simulink model "SG_RaibertControlMonopod"  (R2022a)
settings: Solver=ode4  StartTime=0.0  StopTime=inf  FixedStep=1/4000  MaxStep=0.001  RelTol=1e-3  AbsTol=1e-3  EnableMultiTasking=on
values from neighbouring files (symbols this model uses):
  alternate_legs = InitConstants.alternate_legs    [Controller.m]    (also in ControllerV2.m; ControllerV3.m; Controller_original.m; initialization.m = 1)
  dphi_IC = InitConstants.dphi_IC    [Controller.m]    (also in ControllerV2.m; ControllerV3.m; Controller_original.m; initialization.m = 0)
  dphi_RC_14 = 0.0    (= 0)    [initialization.m]
  dphi_RC_23 = 0.0    (= 0)    [initialization.m]
  dr_contact = -0.2    [initialization.m]
  dr_IC = InitConstants.dr_IC    [Controller.m]    (also in ControllerV2.m; ControllerV3.m; Controller_original.m; initialization.m = 0)
  dr_RC_14 = 0.0    (= 0)    [initialization.m]
  dr_RC_23 = 0.0    (= 0)    [initialization.m]
  dx_des = -InitConstants.dx_des    [Controller.m]    (also in ControllerV2.m; ControllerV3.m; Controller_original.m; Hopper_raibert_controller.m = -min(max(1.0*(x_body - x_des), -0.5), 0.5))
  Fthrust_RC_14 = 100    [initialization.m]
  Fthrust_RC_23 = 150    [initialization.m]
  GAIN_dx_RC_14 = 0.07    [initialization.m]
  GAIN_dx_RC_23 = 0.05    [initialization.m]
  Kd_phi_IC = InitConstants.Kd_phi_IC    [Controller.m]    (also in ControllerV2.m; ControllerV3.m; Controller_original.m; initialization.m = 15)
  Kd_phi_RC_14 = Kp_phi_RC_14*0.1    (= 10)    [initialization.m]
  Kd_phi_RC_23 = 15    [initialization.m]
  Kd_r_IC = InitConstants.Kd_r_IC    [Controller.m]    (also in ControllerV2.m; ControllerV3.m; Controller_original.m; initialization.m = 60)
  Kd_r_RC_14 = Kp_r_RC_14*0.1    (= 60)    [initialization.m]
  Kd_r_RC_23 = 150    [initialization.m]
  knee_limit = 160    [initialization.m]
  Kp_phi_IC = InitConstants.Kp_phi_IC    [Controller.m]    (also in ControllerV2.m; ControllerV3.m; Controller_original.m; initialization.m = 100)
  Kp_phi_RC_14 = 100    [initialization.m]
  Kp_phi_RC_23 = 100    [initialization.m]
  Kp_r_IC = InitConstants.Kp_r_IC    [Controller.m]    (also in ControllerV2.m; ControllerV3.m; Controller_original.m; initialization.m = 500)
  Kp_r_RC_14 = 600    [initialization.m]
  Kp_r_RC_23 = 600    [initialization.m]
  m_eff = 5    [ControllerV2.m]    (also in Controller_original.m; initialization.m)
  match_leg_gains = -1    [initialization.m]
  offset_phi_limit = 30    [initialization.m]
  phi_IC = InitConstants.phi_IC    [Controller.m]    (also in ControllerV2.m; ControllerV3.m; Controller_original.m; initialization.m = 0)
  phi_RC_14 = -0.003    [initialization.m]
  phi_RC_23 = -0.006    [initialization.m]
  r_IC = InitConstants.r_IC    [Controller.m]    (also in ControllerV2.m; ControllerV3.m; Controller_original.m; initialization.m = 0.32)
  r_RC_14 = 0.32    [initialization.m]
  r_RC_23 = 0.33    [initialization.m]
  r_thrust_RC_14 = 0.27    [initialization.m]
  r_thrust_RC_23 = 0.29    [initialization.m]
  tau_limit = 100    [initialization.m]
  update_controller_Kd_r = 1    [initialization.m]
  x_des = InitConstants.x_des    [Controller.m]    (also in ControllerV2.m; ControllerV3.m; Controller_original.m; initialization.m = 0)
undefined symbols (not defined in the file or in its folder): HS, IO291
libraries: speedgoatlib_IO691 x7, canmsglib x5, aru_toolbox x2, simulink x2, speedgoatlib_IO291 x1
(part 2 of 2)

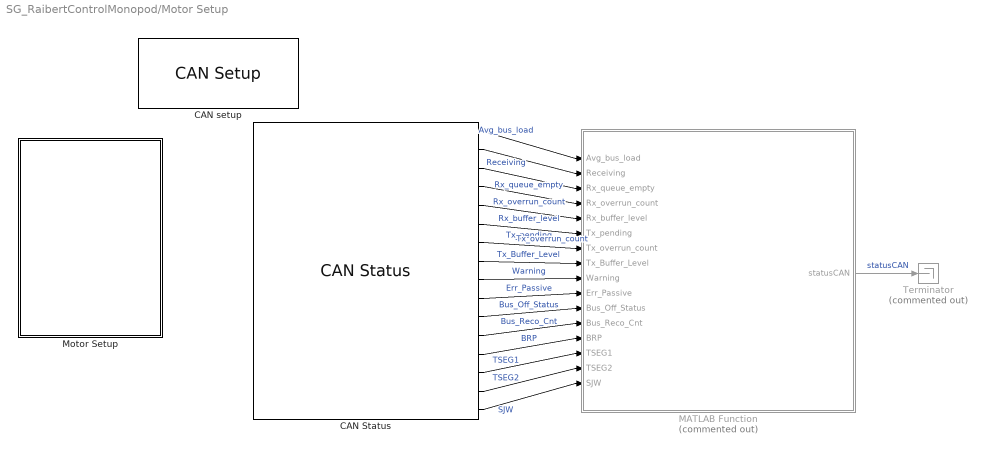
== system SG_RaibertControlMonopod/Motor Setup ==
  CAN Status : speedgoatlib_IO691/Legacy/CAN Status  moduleId=1  sampleTime=-1  channel=1  busRecovery=Off  arrayOutput=off  controllerCpuLoad=off  controllerLiveCount=off  initModeAct=off  avgBusLoad=on  receiving=on  RxQueueEmpty=on  dataOverrunRcv=on  rxBufferLevel=on  txPending=on  dataOverrunTx=on  txBufferLevel=on  errWarnLimit=on  errPassLimit=on  errBusOff=on  busRecoveryCounter=on  busCouplingErr=off  transceiverErr=off  opMode=off  brp=on  timeSegment1=on  timeSegment2=on  synchronisationJumpWidth=on  dataTSEG1=off  dataTSEG2=off  dataSJW=off  moduleType=691  qtyStatBlk=1  ptIdx=0  isFDMod=0
      settings: SourceProductName=Simulink Real-Time: Speedgoat I/O Blockset
  CAN setup : speedgoatlib_IO691/Legacy/CAN Setup   moduletype=IO691  id=1  pciSlot=-1  chn1=CAN (HS)  chn2=Disabled  chn3=Disabled  chn4=Disabled  initStruct=[]  termStruct=[struct('Channel',1,'Protocol','CAN','BRS',0,'Type','Standard','Identifier',2,'Data',[255, 255, 255, 255, 255, 255, 255, 253],'Pause',0.001), struct('Channel',1,'Protocol','CAN','BRS',0,'Type','Standard','Identifier',3,'Data',[255, 255, 255, 255, 255, 255, 255, 253],'Pause',0.001)]  ArbitrationbdrChn1=1.0 MBaud  ArbitrationManbdrChn1=[2,8,31,8]  FdbdrChn1=1.0 MBaud  FdManbdrChn1=[2,8,31,8]  ArbitrationbdrChn2=1.0 MBaud  ArbitrationManbdrChn2=[2,8,31,8]  FdbdrChn2=1.0 MBaud  FdManbdrChn2=[2,8,31,8]  ArbitrationbdrChn3=1.0 MBaud  ArbitrationManbdrChn3=[2,8,31,8]  FdbdrChn3=5.0 MBaud  FdManbdrChn3=[2,2,5,2]  ArbitrationbdrChn4=1.0 MBaud  ArbitrationManbdrChn4=[2,8,31,8]  FdbdrChn4=5.0 MBaud  FdManbdrChn4=[2,2,5,2]  moduleInitValues=[691 1 -1 -1]
      settings: SourceProductName=Simulink Real-Time: Speedgoat I/O Blockset
  MATLAB Function : MATLAB Function  Commented=on  TreatAsAtomicUnit=on
  Motor Setup : Subsystem
  Terminator : Terminator  Commented=on
  wires:
  CAN Status/1 -> MATLAB Function/1(Avg_bus_load)  "Avg_bus_load"
  CAN Status/2 -> MATLAB Function/2(Receiving)  "Receiving"
  CAN Status/3 -> MATLAB Function/3(Rx_queue_empty)  "Rx_queue_empty"
  CAN Status/4 -> MATLAB Function/4(Rx_overrun_count)  "Rx_overrun_count"
  CAN Status/5 -> MATLAB Function/5(Rx_buffer_level)  "Rx_buffer_level"
  CAN Status/6 -> MATLAB Function/6(Tx_pending)  "Tx_pending"
  CAN Status/8 -> MATLAB Function/8(Tx_Buffer_Level)  "Tx_Buffer_Level"
  CAN Status/7 -> MATLAB Function/7(Tx_overrun_count)  "Tx_overrun_count"
  CAN Status/12 -> MATLAB Function/12(Bus_Reco_Cnt)  "Bus_Reco_Cnt"
  CAN Status/13 -> MATLAB Function/13(BRP)  "BRP"
  CAN Status/15 -> MATLAB Function/15(TSEG2)  "TSEG2"
  CAN Status/14 -> MATLAB Function/14(TSEG1)  "TSEG1"
  CAN Status/10 -> MATLAB Function/10(Err_Passive)  "Err_Passive"
  CAN Status/9 -> MATLAB Function/9(Warning)  "Warning"
  CAN Status/11 -> MATLAB Function/11(Bus_Off_Status)  "Bus_Off_Status"
  CAN Status/16 -> MATLAB Function/16(SJW)  "SJW"
  MATLAB Function/1(statusCAN) -> Terminator/1  "statusCAN"

== system SG_RaibertControlMonopod/RC ==
  Trigger : TriggerPort  VariantControl=(inherit)
  Constant : Constant  Value=3
  Out1 : Outport
  wires:
  Constant/1 -> Out1/1

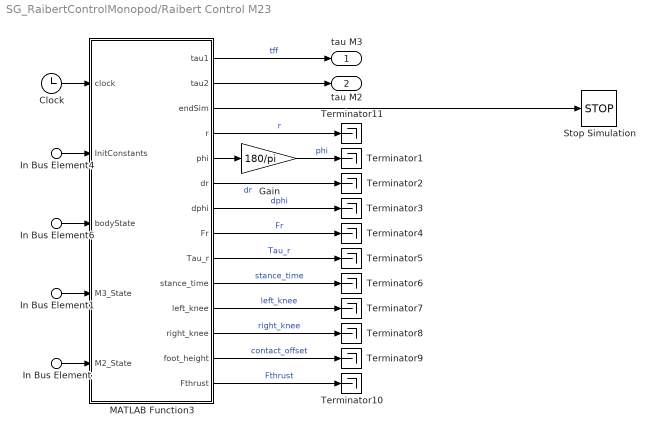
== system SG_RaibertControlMonopod/Raibert Control M23 ==
  In Bus Element4 : Inport  PortName=InitConstants
  In Bus Element6 : Inport  Port=2  PortName=bodyState
  In Bus Element1 : Inport  Port=3  PortName=M3_State
  In Bus Element : Inport  Port=4  PortName=M2_State
  Clock : Clock
  Gain : Gain  Gain=180/pi
  MATLAB Function3 : MATLAB Function  TreatAsAtomicUnit=on
  Stop Simulation : Stop
  Terminator{1..11} (11 alike) : Terminator
  tau M3 : Outport
  tau M2 : Outport  Port=2
  wires:
  In Bus Element6/1 -> MATLAB Function3/3(bodyState)
  In Bus Element/1 -> MATLAB Function3/5(M2_State)
  In Bus Element1/1 -> MATLAB Function3/4(M3_State)
  In Bus Element4/1 -> MATLAB Function3/2(InitConstants)
  Clock/1 -> MATLAB Function3/1(clock)
  MATLAB Function3/3(endSim) -> Stop Simulation/1
  MATLAB Function3/1(tau1) -> tau M3/1  "tff"
  MATLAB Function3/2(tau2) -> tau M2/1
  Gain/1 -> Terminator1/1  "phi"
  MATLAB Function3/4(r) -> Terminator11/1  "r"
  MATLAB Function3/10(stance_time) -> Terminator6/1  "stance_time"
  MATLAB Function3/9(Tau_r) -> Terminator5/1  "Tau_r"
  MATLAB Function3/7(dphi) -> Terminator3/1  "dphi"
  MATLAB Function3/8(Fr) -> Terminator4/1  "Fr"
  MATLAB Function3/6(dr) -> Terminator2/1  "dr"
  MATLAB Function3/11(left_knee) -> Terminator7/1  "left_knee"
  MATLAB Function3/12(right_knee) -> Terminator8/1  "right_knee"
  MATLAB Function3/5(phi) -> Gain/1
  MATLAB Function3/13(foot_height) -> Terminator9/1  "contact_offset"
  MATLAB Function3/14(Fthrust) -> Terminator10/1  "Fthrust"

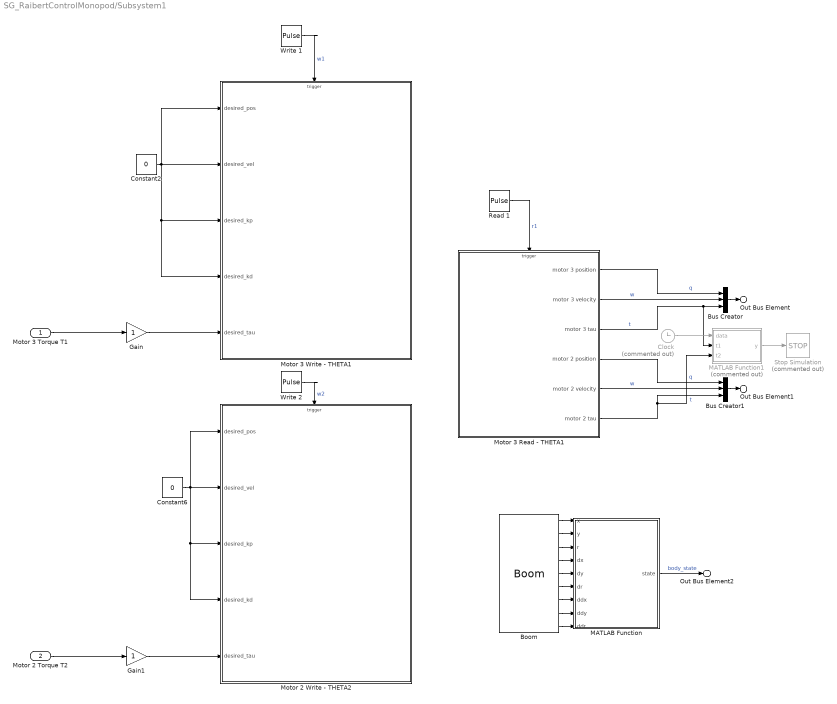
== system SG_RaibertControlMonopod/Subsystem1 ==
  Motor 3 Torque T1 : Inport
  Motor 2 Torque T2 : Inport  Port=2
  Boom : aru_toolbox/Boom  ts=0.001
      link override Serial Read HW FIFO: pciSlot=-1
      link override Serial Setup: pciSlot=-1
      settings: SourceProductName=ARU Toolbox
  Bus Creator : BusCreator  Inputs=3  OutDataTypeStr=Bus: MotorState
  Bus Creator1 : BusCreator  Inputs=3  OutDataTypeStr=Bus: MotorState
  Clock : Clock  Commented=on
  Constant2 : Constant  Value=0
  Constant6 : Constant  Value=0
  Gain : Gain
  Gain1 : Gain
  MATLAB Function : MATLAB Function  TreatAsAtomicUnit=on
  MATLAB Function1 : MATLAB Function  Commented=on  TreatAsAtomicUnit=on
  Motor 2 Write - THETA2 : Subsystem  TreatAsAtomicUnit=on
  Motor 3 Read - THETA1 : Subsystem
  Motor 3 Write - THETA1 : Subsystem  TreatAsAtomicUnit=on
  Read 1 : DiscretePulseGenerator  PulseType=Time based  Period=1/1000  PulseWidth=50  PhaseDelay=3.00025
  Stop Simulation : Stop  Commented=on
  Write 1 : DiscretePulseGenerator  PulseType=Time based  Period=1/1000  PulseWidth=50  PhaseDelay=3
  Write 2 : DiscretePulseGenerator  PulseType=Time based  Period=1/1000  PulseWidth=50  PhaseDelay=3+(1/2000)
  Out Bus Element2 : Outport  PortName=boom state
  Out Bus Element : Outport  Port=2  VectorParamsAs1DForOutWhenUnconnected=off  PortName=M3_State
  Out Bus Element1 : Outport  Port=3  VectorParamsAs1DForOutWhenUnconnected=off  PortName=M2_State
  wires:
  Write 1/1 -> Motor 3 Write - THETA1/Trigger  "w1"
  Read 1/1 -> Motor 3 Read - THETA1/Trigger  "r1"
  Write 2/1 -> Motor 2 Write - THETA2/Trigger  "w2"
  Motor 3 Torque T1/1 -> Gain/1
  Constant6/1 -> Motor 2 Write - THETA2/4(desired_kd), Motor 2 Write - THETA2/3(desired_kp), Motor 2 Write - THETA2/1(desired_pos), Motor 2 Write - THETA2/2(desired_vel)
  Motor 2 Torque T2/1 -> Gain1/1
  Constant2/1 -> Motor 3 Write - THETA1/1(desired_pos), Motor 3 Write - THETA1/4(desired_kd), Motor 3 Write - THETA1/3(desired_kp), Motor 3 Write - THETA1/2(desired_vel)
  Motor 3 Read - THETA1/2(motor 3 velocity) -> Bus Creator/2  "w"
  Motor 3 Read - THETA1/3(motor 3 tau) -> MATLAB Function1/2(t1), Bus Creator/3  "t"
  Bus Creator/1 -> Out Bus Element/1
  Motor 3 Read - THETA1/1(motor 3 position) -> Bus Creator/1  "q"
  Motor 3 Read - THETA1/5(motor 2 velocity) -> Bus Creator1/2  "w"
  Bus Creator1/1 -> Out Bus Element1/1
  Motor 3 Read - THETA1/4(motor 2 position) -> Bus Creator1/1  "q"
  Motor 3 Read - THETA1/6(motor 2 tau) -> MATLAB Function1/3(t2), Bus Creator1/3  "t"
  MATLAB Function/1(state) -> Out Bus Element2/1  "body_state"
  Boom/1 -> MATLAB Function/1(x)
  Boom/2 -> MATLAB Function/2(y)
  Boom/3 -> MATLAB Function/3(r)
  Boom/4 -> MATLAB Function/4(dx)
  Boom/5 -> MATLAB Function/5(dy)
  Boom/6 -> MATLAB Function/6(dr)
  Boom/7 -> MATLAB Function/7(ddx)
  Boom/8 -> MATLAB Function/8(ddy)
  Boom/9 -> MATLAB Function/9(ddr)
  Gain/1 -> Motor 3 Write - THETA1/5(desired_tau)
  Gain1/1 -> Motor 2 Write - THETA2/5(desired_tau)
  MATLAB Function1/1(y) -> Stop Simulation/1
  Clock/1 -> MATLAB Function1/1(data)

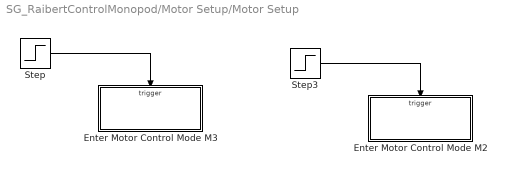
== system SG_RaibertControlMonopod/Motor Setup/Motor Setup ==
  Enter Motor Control Mode M2 : Subsystem  TreatAsAtomicUnit=on
  Enter Motor Control Mode M3 : Subsystem  TreatAsAtomicUnit=on
  Step : Step  Time=1.0
  Step3 : Step  Time=2
  wires:
  Step3/1 -> Enter Motor Control Mode M2/Trigger
  Step/1 -> Enter Motor Control Mode M3/Trigger

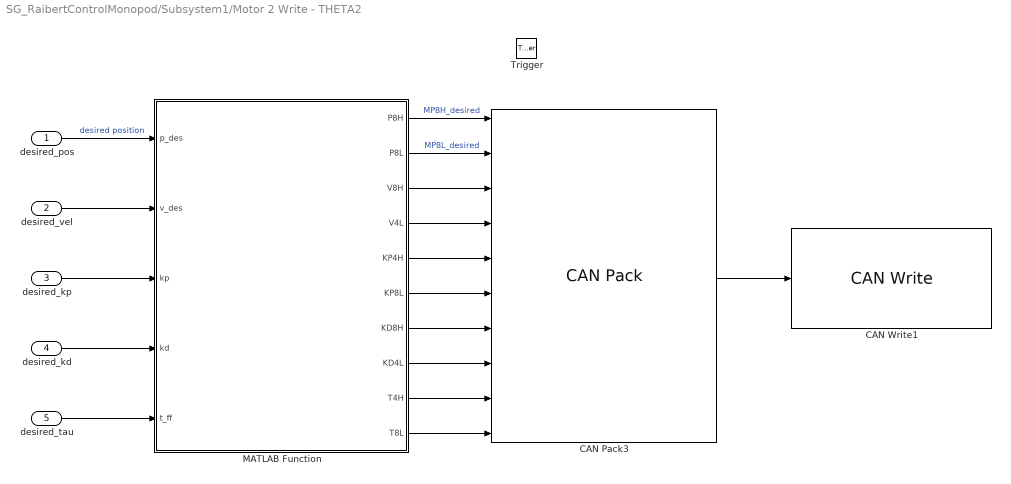
== system SG_RaibertControlMonopod/Subsystem1/Motor 2 Write - THETA2 ==
  desired_pos : Inport
  desired_vel : Inport  Port=2
  desired_kp : Inport  Port=3
  desired_kd : Inport  Port=4
  desired_tau : Inport  Port=5
  Trigger : TriggerPort  VariantControl=Variant
  CAN Pack3 : canmsglib/CAN Pack  MsgList=(none)  MsgName=MotorControl  MsgIDType=Standard (11-bit identifier)  MsgIdentifier=2  MsgLength=8  Remote=off  ApplyMinMax=off  BusOutput=off  SignalInfo={ 'Motor postition 8-H', '0', '8', 'LE', 'unsigned', 'Standard', '0', '1', '0', '-Inf', 'Inf'; 'Motor position 8-L', '8', '8', 'LE', 'unsigned', 'Standard', '0', '1', '0', '-Inf', 'Inf'; 'Motor speed 8-H', '16', '8', 'LE', 'unsigned', 'Standard', '0', '1', '0', '-Inf', 'Inf'; 'Motor speed 4-L', '28', '4', 'LE', 'unsigned', 'Standard', '0', '1', '0', '-Inf', 'Inf'; 'KP 4-H', '24', '4', 'LE', 'unsigned', 'Standard', '0', '1', '0', '-Inf', 'Inf'; 'KP 8-L', '32', '8', 'LE', 'unsigned', 'Standard', '0', '1', '0', '-Inf', 'Inf'; 'KD 8-H', '40', '8', 'LE', 'unsigned', 'Standard', '0', '1', '0', '-Inf', 'Inf'; 'KD 4-L', '52', '4', 'LE', 'unsigned', 'Standard', '0', '1', '0', '-Inf', 'Inf'; 'Current 4-H', '48', '4', 'LE', 'unsigned', 'Standard', '0', '1', '0', '-Inf', 'Inf'; 'Current 8-L', '56', '8', 'LE', 'unsigned', 'Standard', '0', '1', '0', '-Inf', 'Inf' }
      settings: SourceProductBaseCode=XP,ME,VN  DataFormat=manually specified signals
  CAN Write1 : speedgoatlib_IO691/Legacy/CAN Write  id=1  ts=-1  channel=1  messageType=CAN  BusInput=off  enableStatusPort=off  canType=CAN (HS)  initValues=[691 1 -1 0 1 1 0 0]
      settings: SourceProductName=Simulink Real-Time: Speedgoat Library
  MATLAB Function : MATLAB Function  TreatAsAtomicUnit=on
  wires:
  desired_vel/1 -> MATLAB Function/2(v_des)
  desired_pos/1 -> MATLAB Function/1(p_des)  "desired position"
  MATLAB Function/6(KP8L) -> CAN Pack3/6
  MATLAB Function/7(KD8H) -> CAN Pack3/7
  MATLAB Function/2(P8L) -> CAN Pack3/2  "MP8L_desired"
  desired_kp/1 -> MATLAB Function/3(kp)
  MATLAB Function/5(KP4H) -> CAN Pack3/5
  desired_kd/1 -> MATLAB Function/4(kd)
  desired_tau/1 -> MATLAB Function/5(t_ff)
  MATLAB Function/8(KD4L) -> CAN Pack3/8
  MATLAB Function/4(V4L) -> CAN Pack3/4
  MATLAB Function/9(T4H) -> CAN Pack3/9
  MATLAB Function/1(P8H) -> CAN Pack3/1  "MP8H_desired"
  CAN Pack3/1 -> CAN Write1/1
  MATLAB Function/3(V8H) -> CAN Pack3/3
  MATLAB Function/10(T8L) -> CAN Pack3/10

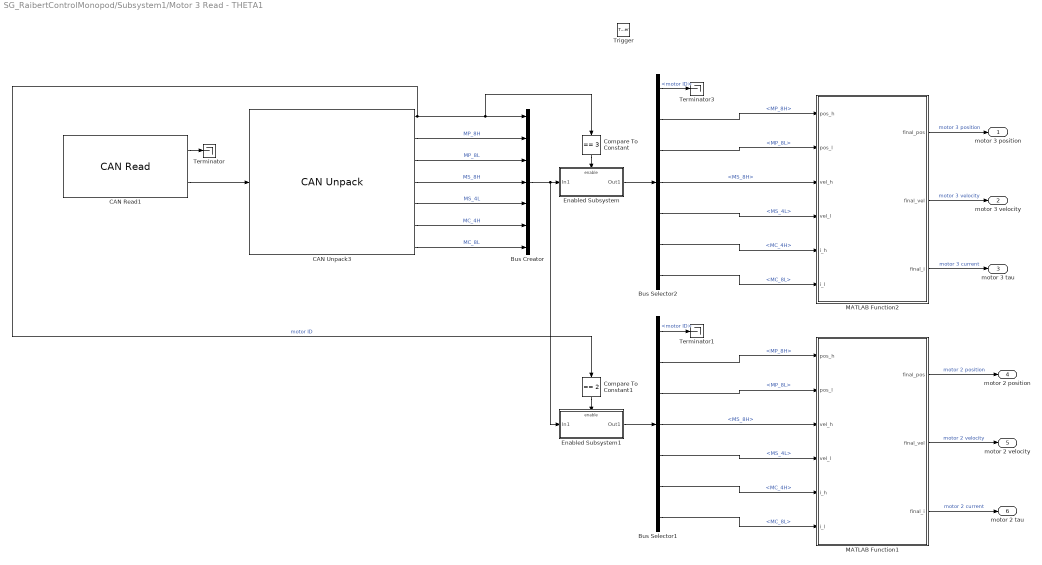
== system SG_RaibertControlMonopod/Subsystem1/Motor 3 Read - THETA1 ==
  Trigger : TriggerPort  TriggerType=either  VariantControl=Variant  PortDimensions=1
  Bus Creator : BusCreator  Inputs=7
  Bus Selector1 : BusSelector  OutputSignals=motor ID,MP_8H,MP_8L,MS_8H,MS_4L,MC_4H,MC_8L
  Bus Selector2 : BusSelector  OutputSignals=motor ID,MP_8H,MP_8L,MS_8H,MS_4L,MC_4H,MC_8L
  CAN Read1 : speedgoatlib_IO691/Legacy/CAN Read  id=1  ts=-1  channel=1  messageType=CAN  canType=CAN (HS)  BusOutput=off  initValues=[691 1 -1 0 1 1 0]
      settings: SourceProductName=Simulink Real-Time: Speedgoat Library
  CAN Unpack3 : canmsglib/CAN Unpack  MsgList=(none)  MsgName=CAN Msg  MsgIDType=Standard (11-bit identifier)  MsgIdentifier=0  MsgLength=8  SignalInfo={ 'Drive ID', '0', '8', 'LE', 'unsigned', 'Standard', '0', '1', '0', '-Inf', 'Inf'; 'Motor position 8-H', '8', '8', 'LE', 'unsigned', 'Standard', '0', '1', '0', '-Inf', 'Inf'; 'Motor position 8-L', '16', '8', 'LE', 'unsigned', 'Standard', '0', '1', '0', '-Inf', 'Inf'; 'Motor speed 8-H', '24', '8', 'LE', 'unsigned', 'Standard', '0', '1', '0', '-Inf', 'Inf'; 'Motor speed 4-L', '36', '4', 'LE', 'unsigned', 'Standard', '0', '1', '0', '-Inf', 'Inf'; 'Current 4-H', '32', '4', 'LE', 'unsigned', 'Standard', '0', '1', '0', '-Inf', 'Inf'; 'Current 8-L', '40', '8', 'LE', 'unsigned', 'Standard', '0', '1', '0', '-Inf', 'Inf' }  IDPort=off  TimestampPort=off  ErrorPort=off  RemotePort=off  LengthPort=off  StatusPort=off  ApplyMinMax=off
      settings: SourceProductBaseCode=XP,ME,VN
  Compare To Constant : simulink/Logic and Bit Operations/Compare To Constant  relop===  const=3  OutDataTypeStr=boolean
  Compare To Constant1 : simulink/Logic and Bit Operations/Compare To Constant  relop===  const=2  OutDataTypeStr=boolean
  Enabled Subsystem : Subsystem  TreatAsAtomicUnit=on
  Enabled Subsystem1 : Subsystem  TreatAsAtomicUnit=on
  MATLAB Function1 : MATLAB Function  TreatAsAtomicUnit=on
  MATLAB Function2 : MATLAB Function  TreatAsAtomicUnit=on
  Terminator : Terminator
  Terminator1 : Terminator
  Terminator3 : Terminator
  motor 3 position : Outport
  motor 3 velocity : Outport  Port=2
  motor 3 tau : Outport  Port=3
  motor 2 position : Outport  Port=4
  motor 2 velocity : Outport  Port=5
  motor 2 tau : Outport  Port=6
  wires:
  MATLAB Function2/3(final_i) -> motor 3 tau/1  "motor 3 current"
  MATLAB Function2/1(final_pos) -> motor 3 position/1  "motor 3 position"
  MATLAB Function2/2(final_vel) -> motor 3 velocity/1  "motor 3 velocity"
  CAN Unpack3/7 -> Bus Creator/7  "MC_8L"
  Bus Selector2/4 -> MATLAB Function2/3(vel_h)  "<MS_8H>"
  Bus Selector2/7 -> MATLAB Function2/6(i_l)  "<MC_8L>"
  CAN Unpack3/4 -> Bus Creator/4  "MS_8H"
  CAN Unpack3/6 -> Bus Creator/6  "MC_4H"
  Bus Selector2/1 -> Terminator3/1  "<motor ID>"
  CAN Unpack3/3 -> Bus Creator/3  "MP_8L"
  Bus Selector2/2 -> MATLAB Function2/1(pos_h)  "<MP_8H>"
  Bus Selector2/5 -> MATLAB Function2/4(vel_l)  "<MS_4L>"
  CAN Unpack3/2 -> Bus Creator/2  "MP_8H"
  CAN Read1/2 -> CAN Unpack3/1
  CAN Unpack3/5 -> Bus Creator/5  "MS_4L"
  Bus Selector2/6 -> MATLAB Function2/5(i_h)  "<MC_4H>"
  Bus Selector2/3 -> MATLAB Function2/2(pos_l)  "<MP_8L>"
  Compare To Constant/1 -> Enabled Subsystem/Enable
  Bus Creator/1 -> Enabled Subsystem1/1(In1), Enabled Subsystem/1(In1)
  Enabled Subsystem/1(Out1) -> Bus Selector2/1
  CAN Read1/1 -> Terminator/1
  CAN Unpack3/1 -> Bus Creator/1, Compare To Constant/1, Compare To Constant1/1  "motor ID"
  Bus Selector1/2 -> MATLAB Function1/1(pos_h)  "<MP_8H>"
  Compare To Constant1/1 -> Enabled Subsystem1/Enable
  Bus Selector1/6 -> MATLAB Function1/5(i_h)  "<MC_4H>"
  Enabled Subsystem1/1(Out1) -> Bus Selector1/1
  Bus Selector1/3 -> MATLAB Function1/2(pos_l)  "<MP_8L>"
  Bus Selector1/5 -> MATLAB Function1/4(vel_l)  "<MS_4L>"
  MATLAB Function1/1(final_pos) -> motor 2 position/1  "motor 2 position"
  Bus Selector1/1 -> Terminator1/1  "<motor ID>"
  MATLAB Function1/2(final_vel) -> motor 2 velocity/1  "motor 2 velocity"
  MATLAB Function1/3(final_i) -> motor 2 tau/1  "motor 2 current"
  Bus Selector1/4 -> MATLAB Function1/3(vel_h)  "<MS_8H>"
  Bus Selector1/7 -> MATLAB Function1/6(i_l)  "<MC_8L>"

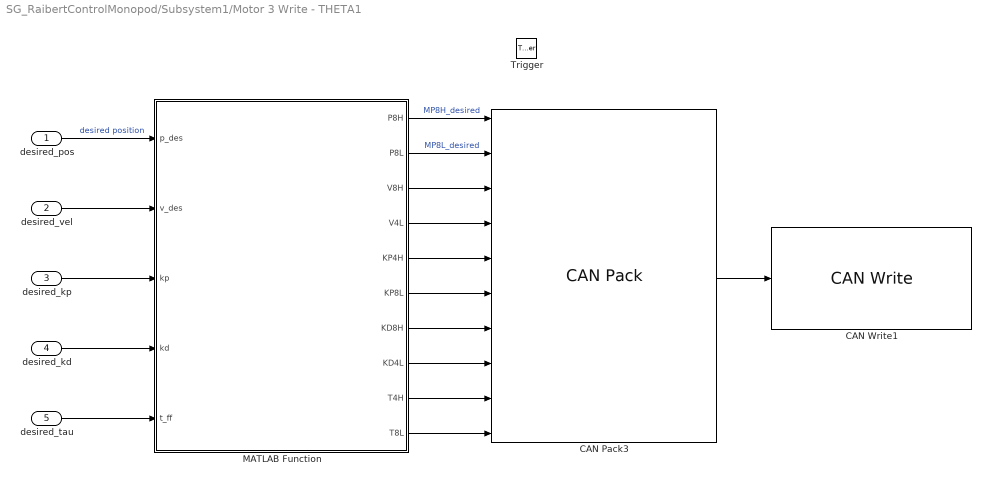
== system SG_RaibertControlMonopod/Subsystem1/Motor 3 Write - THETA1 ==
  desired_pos : Inport
  desired_vel : Inport  Port=2
  desired_kp : Inport  Port=3
  desired_kd : Inport  Port=4
  desired_tau : Inport  Port=5
  Trigger : TriggerPort  VariantControl=Variant
  CAN Pack3 : canmsglib/CAN Pack  MsgList=(none)  MsgName=MotorControl  MsgIDType=Standard (11-bit identifier)  MsgIdentifier=3  MsgLength=8  Remote=off  ApplyMinMax=off  BusOutput=off  SignalInfo={ 'Motor postition 8-H', '0', '8', 'LE', 'unsigned', 'Standard', '0', '1', '0', '-Inf', 'Inf'; 'Motor position 8-L', '8', '8', 'LE', 'unsigned', 'Standard', '0', '1', '0', '-Inf', 'Inf'; 'Motor speed 8-H', '16', '8', 'LE', 'unsigned', 'Standard', '0', '1', '0', '-Inf', 'Inf'; 'Motor speed 4-L', '28', '4', 'LE', 'unsigned', 'Standard', '0', '1', '0', '-Inf', 'Inf'; 'KP 4-H', '24', '4', 'LE', 'unsigned', 'Standard', '0', '1', '0', '-Inf', 'Inf'; 'KP 8-L', '32', '8', 'LE', 'unsigned', 'Standard', '0', '1', '0', '-Inf', 'Inf'; 'KD 8-H', '40', '8', 'LE', 'unsigned', 'Standard', '0', '1', '0', '-Inf', 'Inf'; 'KD 4-L', '52', '4', 'LE', 'unsigned', 'Standard', '0', '1', '0', '-Inf', 'Inf'; 'Current 4-H', '48', '4', 'LE', 'unsigned', 'Standard', '0', '1', '0', '-Inf', 'Inf'; 'Current 8-L', '56', '8', 'LE', 'unsigned', 'Standard', '0', '1', '0', '-Inf', 'Inf' }
      settings: SourceProductBaseCode=XP,ME,VN  DataFormat=manually specified signals
  CAN Write1 : speedgoatlib_IO691/Legacy/CAN Write  id=1  ts=-1  channel=1  messageType=CAN  BusInput=off  enableStatusPort=off  canType=CAN (HS)  initValues=[691 1 -1 0 1 1 0 0]
      settings: SourceProductName=Simulink Real-Time: Speedgoat I/O Blockset
  MATLAB Function : MATLAB Function  TreatAsAtomicUnit=on
  wires:
  desired_vel/1 -> MATLAB Function/2(v_des)
  desired_pos/1 -> MATLAB Function/1(p_des)  "desired position"
  MATLAB Function/6(KP8L) -> CAN Pack3/6
  MATLAB Function/7(KD8H) -> CAN Pack3/7
  MATLAB Function/2(P8L) -> CAN Pack3/2  "MP8L_desired"
  desired_kp/1 -> MATLAB Function/3(kp)
  MATLAB Function/5(KP4H) -> CAN Pack3/5
  desired_kd/1 -> MATLAB Function/4(kd)
  desired_tau/1 -> MATLAB Function/5(t_ff)
  MATLAB Function/8(KD4L) -> CAN Pack3/8
  MATLAB Function/4(V4L) -> CAN Pack3/4
  MATLAB Function/9(T4H) -> CAN Pack3/9
  MATLAB Function/1(P8H) -> CAN Pack3/1  "MP8H_desired"
  CAN Pack3/1 -> CAN Write1/1
  MATLAB Function/3(V8H) -> CAN Pack3/3
  MATLAB Function/10(T8L) -> CAN Pack3/10

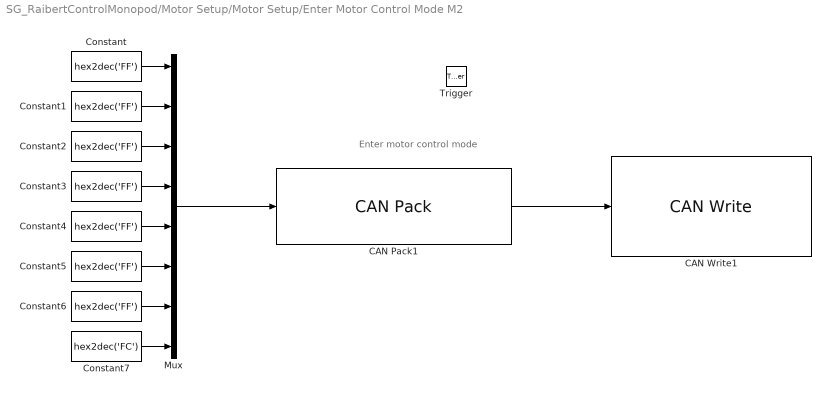
== system SG_RaibertControlMonopod/Motor Setup/Motor Setup/Enter Motor Control Mode M2 ==
  note: Enter motor control mode
  Trigger : TriggerPort  VariantControl=Variant
  CAN Pack1 : canmsglib/CAN Pack  MsgList=(none)  MsgName=CAN Msg  MsgIDType=Standard (11-bit identifier)  MsgIdentifier=2  MsgLength=8  Remote=off  ApplyMinMax=off  BusOutput=off  SignalInfo={ 'Motor postition 8-H', '0', '8', 'LE', 'unsigned', 'Standard', '0', '1', '0', '-Inf', 'Inf'; 'Motor position 8-L', '8', '8', 'LE', 'unsigned', 'Standard', '0', '1', '0', '-Inf', 'Inf'; 'Motor seed 8-H', '16', '8', 'LE', 'unsigned', 'Standard', '0', '1', '0', '-Inf', 'Inf'; 'Motor speed 4-L', '28', '4', 'LE', 'unsigned', 'Standard', '0', '1', '0', '-Inf', 'Inf'; 'KP 4-H', '24', '4', 'LE', 'unsigned', 'Standard', '0', '1', '0', '-Inf', 'Inf'; 'KP 8-L', '32', '8', 'LE', 'unsigned', 'Standard', '0', '1', '0', '-Inf', 'Inf'; 'KP 8-H', '40', '8', 'LE', 'unsigned', 'Standard', '0', '1', '0', '-Inf', 'Inf'; 'KD 4-L', '52', '4', 'LE', 'unsigned', 'Standard', '0', '1', '0', '-Inf', 'Inf'; 'Current 4-H', '48', '4', 'LE', 'unsigned', 'Standard', '0', '1', '0', '-Inf', 'Inf'; 'Current 8-L', '56', '8', 'LE', 'unsigned', 'Standard', '0', '1', '0', '-Inf', 'Inf' }
      settings: SourceProductBaseCode=ME,XP,VN  DataFormat=raw data
  CAN Write1 : speedgoatlib_IO691/Legacy/CAN Write  id=1  ts=-1  channel=1  messageType=CAN  BusInput=off  enableStatusPort=off  canType=CAN (HS)  initValues=[691 1 -1 0 1 1 0 0]
      settings: SourceProductName=Simulink Real-Time: Speedgoat Library
  Constant{,1..6} (7 alike) : Constant  Value=hex2dec('FF')  OutDataTypeStr=uint8  SampleTime=-1
  Constant7 : Constant  Value=hex2dec('FC')  OutDataTypeStr=uint8  SampleTime=-1
  Mux : Mux  Inputs=8
  wires:
  CAN Pack1/1 -> CAN Write1/1
  Mux/1 -> CAN Pack1/1
  Constant7/1 -> Mux/8
  Constant4/1 -> Mux/5
  Constant1/1 -> Mux/2
  Constant5/1 -> Mux/6
  Constant3/1 -> Mux/4
  Constant2/1 -> Mux/3
  Constant/1 -> Mux/1
  Constant6/1 -> Mux/7

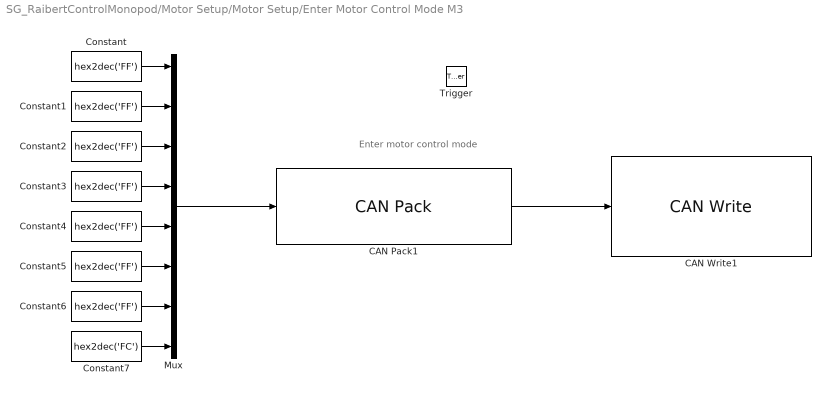
== system SG_RaibertControlMonopod/Motor Setup/Motor Setup/Enter Motor Control Mode M3 ==
  note: Enter motor control mode
  Trigger : TriggerPort  VariantControl=Variant
  CAN Pack1 : canmsglib/CAN Pack  MsgList=(none)  MsgName=CAN Msg  MsgIDType=Standard (11-bit identifier)  MsgIdentifier=3  MsgLength=8  Remote=off  ApplyMinMax=off  BusOutput=off  SignalInfo={ 'Motor postition 8-H', '0', '8', 'LE', 'unsigned', 'Standard', '0', '1', '0', '-Inf', 'Inf'; 'Motor position 8-L', '8', '8', 'LE', 'unsigned', 'Standard', '0', '1', '0', '-Inf', 'Inf'; 'Motor seed 8-H', '16', '8', 'LE', 'unsigned', 'Standard', '0', '1', '0', '-Inf', 'Inf'; 'Motor speed 4-L', '28', '4', 'LE', 'unsigned', 'Standard', '0', '1', '0', '-Inf', 'Inf'; 'KP 4-H', '24', '4', 'LE', 'unsigned', 'Standard', '0', '1', '0', '-Inf', 'Inf'; 'KP 8-L', '32', '8', 'LE', 'unsigned', 'Standard', '0', '1', '0', '-Inf', 'Inf'; 'KP 8-H', '40', '8', 'LE', 'unsigned', 'Standard', '0', '1', '0', '-Inf', 'Inf'; 'KD 4-L', '52', '4', 'LE', 'unsigned', 'Standard', '0', '1', '0', '-Inf', 'Inf'; 'Current 4-H', '48', '4', 'LE', 'unsigned', 'Standard', '0', '1', '0', '-Inf', 'Inf'; 'Current 8-L', '56', '8', 'LE', 'unsigned', 'Standard', '0', '1', '0', '-Inf', 'Inf' }
      settings: SourceProductBaseCode=ME,XP,VN  DataFormat=raw data
  CAN Write1 : speedgoatlib_IO691/Legacy/CAN Write  id=1  ts=-1  channel=1  messageType=CAN  BusInput=off  enableStatusPort=off  canType=CAN (HS)  initValues=[691 1 -1 0 1 1 0 0]
      settings: SourceProductName=Simulink Real-Time: Speedgoat Library
  Constant{,1..6} (7 alike) : Constant  Value=hex2dec('FF')  OutDataTypeStr=uint8  SampleTime=-1
  Constant7 : Constant  Value=hex2dec('FC')  OutDataTypeStr=uint8  SampleTime=-1
  Mux : Mux  Inputs=8
  wires:
  CAN Pack1/1 -> CAN Write1/1
  Mux/1 -> CAN Pack1/1
  Constant7/1 -> Mux/8
  Constant4/1 -> Mux/5
  Constant1/1 -> Mux/2
  Constant5/1 -> Mux/6
  Constant3/1 -> Mux/4
  Constant2/1 -> Mux/3
  Constant/1 -> Mux/1
  Constant6/1 -> Mux/7

== system SG_RaibertControlMonopod/Subsystem1/Motor 3 Read - THETA1/Enabled Subsystem ==
  In1 : Inport
  Enable : EnablePort
  Out1 : Outport
  wires:
  In1/1 -> Out1/1

== system SG_RaibertControlMonopod/Subsystem1/Motor 3 Read - THETA1/Enabled Subsystem1 ==
  In1 : Inport
  Enable : EnablePort
  Out1 : Outport
  wires:
  In1/1 -> Out1/1

== matlab function SG_RaibertControlMonopod/Motor Setup/MATLAB Function ==
  data: Avg_bus_load input; Receiving input; statusCAN output Bus: BodyState; Rx_queue_empty input; Rx_overrun_count input; Rx_buffer_level input; Tx_pending input; Tx_overrun_count input; Tx_Buffer_Level input; Warning input; Err_Passive input; Bus_Off_Status input; Bus_Reco_Cnt input; BRP input; TSEG1 input; TSEG2 input; SJW input
function statusCAN  = CANBUS_state(Avg_bus_load,Receiving,Rx_queue_empty,Rx_overrun_count,Rx_buffer_level,Tx_pending,Tx_overrun_count,Tx_Buffer_Level,Warning,Err_Passive,Bus_Off_Status,Bus_Reco_Cnt,BRP,TSEG1,TSEG2,SJW)
statusCAN.Avg_bus_load = Avg_bus_load;
statusCAN.Receiving = Receiving;
statusCAN.Rx_queue_empty = Rx_queue_empty;
statusCAN.Rx_overrun_count = Rx_overrun_count;
statusCAN.Rx_buffer_level = Rx_buffer_level;
statusCAN.Tx_pending = Tx_pending;
statusCAN.Tx_overrun_count = Tx_overrun_count;
statusCAN.Tx_Buffer_Level = Tx_Buffer_Level;
statusCAN.Warning = Warning;
statusCAN.Err_Passive = Err_Passive;
statusCAN.Bus_Off_Status = Bus_Off_Status;
statusCAN.Bus_Reco_Cnt = Bus_Reco_Cnt;
statusCAN.BRP = BRP;
statusCAN.TSEG1 = TSEG1;
statusCAN.TSEG2 = TSEG2;
statusCAN.SJW = SJW;

end

== matlab function SG_RaibertControlMonopod/Subsystem1/MATLAB Function ==
  data: x input; y input; state output Bus: BodyState; r input; dx input; dy input; dr input; ddx input; ddy input; ddr input
function state  = boom_state(x,y,r,dx,dy,dr,ddx,ddy,ddr)
state.x = x;
state.dx = dx;
state.ddx = ddx;

state.y = y;
state.dy = dy;
state.ddy = ddy;

state.r = r;
state.dr = dr;
end

== matlab function SG_RaibertControlMonopod/Subsystem1/Motor 3 Write - THETA1/MATLAB Function ==
  data: p_des input; P8H output; v_des input; kp input; kd input; t_ff input; P8L output; V8H output; V4L output; KP4H output; KP8L output; KD8H output; KD4L output; T4H output; T8L output
function [P8H,P8L,V8H,V4L,KP4H,KP8L,KD8H,KD4L,T4H,T8L] = AK1090(p_des, v_des, kp, kd, t_ff)
    % Coppied from AK70-10 manual
    % NB: CONSTANTS FOR AK70-10
    p_min = -12.5; % rad
    p_max = +12.5; % rad
    v_min = -50.0; % rad/s
    v_max = +50.0; % rad/s
    t_min = -65.0; % Nm
    t_max = +65.0; % Nm
    kp_min = 0;
    kp_max = 500;
    kd_min = 0;
    kd_max = 5;
    
    % bound inputs
    p_des = min([max([p_min,p_des]),p_max]);
    v_des = min([max([v_min,v_des]),v_max]);
    kp = min([max([kp_min,kp]),kp_max]);
    kd = min([max([kd_min,kd]),kd_max]);
    t_ff = min([max([t_min,t_ff]),t_max]);
    
    % convert floats to unsigned integers
    p_int = float_to_uint(p_des, p_min, p_max, 16);
    v_int = float_to_uint(v_des, v_min, v_max, 12);
    kp_int = float_to_uint(kp, kp_min, kp_max, 12);
    kd_int = float_to_uint(kd, kd_min, kd_max, 12);
    t_int = float_to_uint(t_ff, t_min, t_max, 12);
    
    % break up for CAN frame 
    P8H = bitshift(p_int, -8); % 8 higher bits
    P8L = bitand(p_int, 0xFF); % 8 lower bits
    V8H = bitshift(v_int, -4); % 8 higher bits
    V4L = bitand(v_int, 0xF); % 4 lower bits
    KP4H = bitshift(kp_int, -8); % 4 higher bits
    KP8L = bitand(kp_int, 0xFF); % 8 lower bits
    KD8H = bitshift(kd_int, -4); % 8 higher bits
    KD4L = bitand(kd_int, 0xF); % 4 lower bits
    T4H = bitshift(t_int, -8); % 4 higher bits
    T8L = bitand(t_int, 0xFF); % 8 lower bits
    
    % Converts a float to an unsigned int, given range and number of bits
    function x_int = float_to_uint(x, x_min, x_max, n_bits)
        span = x_max - x_min;
        min([max([x_min,x]),x_max])
        x_int = ((x - x_min)*(bitshift(1, n_bits) / span));
    end
end
%final_values = desired_pos,desired_vel,desired_kp,desired_kd,desired_tau;

== matlab function SG_RaibertControlMonopod/Raibert Control M23/MATLAB Function3 ==
  settings: updateMethod=DISCRETE
  data: clock input; InitConstants input; bodyState input; tau1 output; tau2 output; endSim output; M3_State input; r output; M2_State input; phi output; dr output; dphi output; Fr output; Tau_r output; stance_time output; left_knee output; right_knee output; foot_height output; Fthrust output
function [tau1,tau2,endSim,r,phi,dr,dphi,Fr,Tau_r,stance_time,left_knee,right_knee,foot_height,Fthrust]  = RController(clock,InitConstants,bodyState,M3_State,M2_State)
    motors = 23;
    theta_ML = M3_State.q;
    theta_MR = M2_State.q;
    dtheta_ML = M3_State.w;
    dtheta_MR = M2_State.w;
   
    [B,polarPosition,polarVelocity,Forces,stance_timer,knee_angles,contact_values,endSim] =  Controller(clock,motors,InitConstants,bodyState,theta_ML,theta_MR,dtheta_ML,dtheta_MR);
    tau1 = B(1);
    tau2 = B(2);
    r = polarPosition(1);
    phi = polarPosition(2);
    dr = polarVelocity(1);
    dphi = polarVelocity(2);
    Fr = Forces(1);
    Tau_r = Forces(2);
    stance_time = stance_timer; 
    left_knee = knee_angles(1);
    right_knee = knee_angles(2);
    foot_height = contact_values(2);
    Fthrust = contact_values(1);
    
end

== matlab function SG_RaibertControlMonopod/Subsystem1/Motor 3 Read - THETA1/MATLAB Function2 ==
  data: pos_h input; final_pos output; pos_l input; vel_h input; vel_l input; i_h input; i_l input; final_vel output; final_i output
function [final_pos,final_vel,final_i] = fcn(pos_h,pos_l,vel_h,vel_l,i_h,i_l)
% ------------------------------------
max_pos = 12.5;
min_pos = -12.5;
span_pos = max_pos - min_pos;
offset_pos = max_pos;

pos = bitshift(pos_h,8);
combined_pos = bitor(pos,pos_l);

range_pos = ((combined_pos*span_pos)/(2^16-1))-offset_pos;

final_pos = (range_pos*4*pi)/12.5;
% ------------------------------------
max_vel = 23.24;
min_vel = -23.24;
span_vel = max_vel - min_vel;
offset_vel = max_vel;
vel = bitshift(vel_h,4);
combined_vel = bitor(vel,vel_l);

final_vel = ((combined_vel*span_vel)/(2^12-1))-offset_vel;

% ------------------------------------
max_i = 54;
min_i = -54;
span_i = max_i - min_i;
offset_i = max_i;
i = bitshift(i_h,8);
combined_i = bitor(i,i_l);

final_i = ((combined_i*span_i)/(2^12-1))-offset_i;
end

== matlab function SG_RaibertControlMonopod/Subsystem1/Motor 2 Write - THETA2/MATLAB Function ==
  data: p_des input; P8H output; v_des input; kp input; kd input; t_ff input; P8L output; V8H output; V4L output; KP4H output; KP8L output; KD8H output; KD4L output; T4H output; T8L output
function [P8H,P8L,V8H,V4L,KP4H,KP8L,KD8H,KD4L,T4H,T8L] = AK1090(p_des, v_des, kp, kd, t_ff)
    % Coppied from AK70-10 manual
    % NB: CONSTANTS FOR AK70-10
    p_min = -12.5; % rad
    p_max = +12.5; % rad
    v_min = -50.0; % rad/s
    v_max = +50.0; % rad/s
    t_min = -65.0; % Nm
    t_max = +65.0; % Nm
    kp_min = 0;
    kp_max = 500;
    kd_min = 0;
    kd_max = 5;
    
    % bound inputs
    p_des = min([max([p_min,p_des]),p_max]);
    v_des = min([max([v_min,v_des]),v_max]);
    kp = min([max([kp_min,kp]),kp_max]);
    kd = min([max([kd_min,kd]),kd_max]);
    t_ff = min([max([t_min,t_ff]),t_max]);
    
    % convert floats to unsigned integers
    p_int = float_to_uint(p_des, p_min, p_max, 16);
    v_int = float_to_uint(v_des, v_min, v_max, 12);
    kp_int = float_to_uint(kp, kp_min, kp_max, 12);
    kd_int = float_to_uint(kd, kd_min, kd_max, 12);
    t_int = float_to_uint(t_ff, t_min, t_max, 12);
    
    % break up for CAN frame 
    P8H = bitshift(p_int, -8); % 8 higher bits
    P8L = bitand(p_int, 0xFF); % 8 lower bits
    V8H = bitshift(v_int, -4); % 8 higher bits
    V4L = bitand(v_int, 0xF); % 4 lower bits
    KP4H = bitshift(kp_int, -8); % 4 higher bits
    KP8L = bitand(kp_int, 0xFF); % 8 lower bits
    KD8H = bitshift(kd_int, -4); % 8 higher bits
    KD4L = bitand(kd_int, 0xF); % 4 lower bits
    T4H = bitshift(t_int, -8); % 4 higher bits
    T8L = bitand(t_int, 0xFF); % 8 lower bits
    
    % Converts a float to an unsigned int, given range and number of bits
    function x_int = float_to_uint(x, x_min, x_max, n_bits)
        span = x_max - x_min;
        min([max([x_min,x]),x_max])
        x_int = ((x - x_min)*(bitshift(1, n_bits) / span));
    end
end
%final_values = desired_pos,desired_vel,desired_kp,desired_kd,desired_tau;

== matlab function SG_RaibertControlMonopod/Subsystem1/Motor 3 Read - THETA1/MATLAB Function1 ==
  data: pos_h input; final_pos output; pos_l input; vel_h input; vel_l input; i_h input; i_l input; final_vel output; final_i output
function [final_pos,final_vel,final_i] = fcn(pos_h,pos_l,vel_h,vel_l,i_h,i_l)
% ------------------------------------
max_pos = 12.5;
min_pos = -12.5;
span_pos = max_pos - min_pos;
offset_pos = max_pos;

pos = bitshift(pos_h,8);
combined_pos = bitor(pos,pos_l);

range_pos = ((combined_pos*span_pos)/(2^16-1))-offset_pos;

final_pos = (range_pos*4*pi)/12.5;
% ------------------------------------
max_vel = 23.24;
min_vel = -23.24;
span_vel = max_vel - min_vel;
offset_vel = max_vel;
vel = bitshift(vel_h,4);
combined_vel = bitor(vel,vel_l);

final_vel = ((combined_vel*span_vel)/(2^12-1))-offset_vel;

% ------------------------------------
max_i = 54;
min_i = -54;
span_i = max_i - min_i;
offset_i = max_i;
i = bitshift(i_h,8);
combined_i = bitor(i,i_l);

final_i = ((combined_i*span_i)/(2^12-1))-offset_i;
end

== matlab function SG_RaibertControlMonopod/Subsystem1/MATLAB Function1 ==
  data: data input; t1 input; y output; t2 input
function y = fcn(data, t1,t2)
    if (abs(t1) >10 || abs(t2) >10) && data>4
        y = 1;
    else
        y = 0;
    end
end
